simulink model "adaptive_mdl"  (R2025b)
settings: Solver=ode8  StartTime=0.0  StopTime=150  RelTol=1e-3
undefined symbols (not defined in the file): K, L0, omega, T, Tf, umax
libraries: simulink x2
settings Model: Creator=rapaja  LastModifiedBy=Predrag
settings SolverCC: AlgebraicLoopSolver=TrustRegion
settings DebuggingCC: UnconnectedInputMsg=warning  UnconnectedOutputMsg=warning  UnconnectedLineMsg=warning
settings ModelReferenceCC: EnableRefExpFcnMdlSchedulingChecks=on
settings RTWCC: GPUComputeCapability=3.5

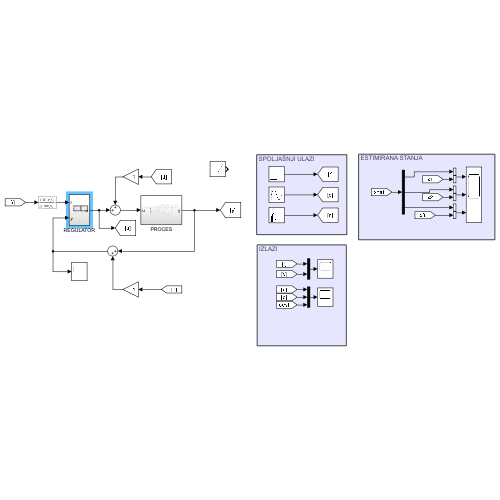
[thumbnail: Simulink's stored preview of the top-level diagram]
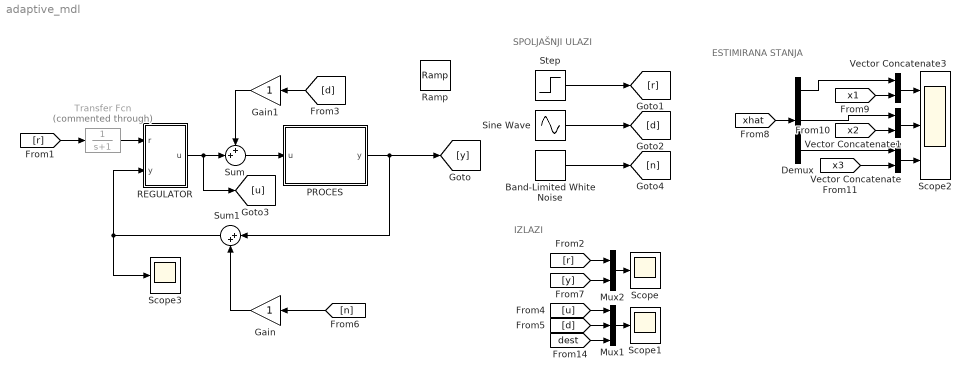
== system adaptive_mdl ==
  note: ESTIMIRANA STANJA
  note: IZLAZI
  note: SPOLJAŠNJI ULAZI
  Band-Limited White Noise : simulink/Sources/Band-Limited White Noise  Cov=[0.00001]  Ts=T  seed=[23341]
  Demux : Demux  Outputs=3
  Gain : Gain
  Gain1 : Gain
  Mux1 : Mux  Inputs=3
  Mux2 : Mux  Inputs=2
  PROCES : Subsystem
  REGULATOR : Subsystem
  Ramp : simulink/Sources/Ramp  slope=1  start=0  InitialOutput=0
  Scope : Scope
      settings: ActiveDisplayYMinimum=-7.6055878064098327E+152  ActiveDisplayYMaximum=1.3812329514646694E+152
  Scope1 : Scope
      settings: ActiveDisplayYMinimum=-4.4199585625146725  ActiveDisplayYMaximum=30.491106506946075
  Scope2 : Scope  NumInputPorts=3
      settings: ActiveDisplayYMinimum=-0.25565847863628133  ActiveDisplayYMaximum=2.1794222293336483  DataLoggingVariableName=ScopeData2
  Scope3 : Scope
      settings: ActiveDisplayYMinimum=-4.0357975554112038  ActiveDisplayYMaximum=7.5925968634709662  DataLoggingVariableName=ScopeData3
  Sine Wave : Sin  Amplitude=0.1  Frequency=omega  SampleTime=0
  Step : Step  Time=2  SampleTime=0
  Sum : Sum  Inputs=++|
  Sum1 : Sum  Inputs=|++
  Transfer Fcn : TransferFcn  Commented=through  Denominator=[1 1]
  Vector Concatenate : Concatenate
  Vector Concatenate1 : Concatenate
  Vector Concatenate3 : Concatenate
  wires:
  REGULATOR/1(u) -> Sum/2, [u]
  [d] -> Gain1/1
  Band-Limited White Noise/1 -> [n]
  Gain/1 -> Sum1/2
  Gain1/1 -> Sum/1
  [r] -> Mux2/1
  [y] -> Mux2/2
  Mux2/1 -> Scope/1
  Mux1/1 -> Scope1/1
  [u] -> Mux1/1
  [d] -> Mux1/2
  PROCES/1(y) -> Sum1/1, [y]
  Sum/1 -> PROCES/1(u)
  Sum1/1 -> Scope3/1, REGULATOR/2(y)
  Step/1 -> [r]
  [n] -> Gain/1
  [r] -> Transfer Fcn/1
  [xhat] -> Demux/1
  Vector Concatenate/1 -> Scope2/3
  Demux/3 -> Vector Concatenate/1
  [x3] -> Vector Concatenate/2
  Vector Concatenate1/1 -> Scope2/2
  Demux/2 -> Vector Concatenate1/1
  [x2] -> Vector Concatenate1/2
  Vector Concatenate3/1 -> Scope2/1
  [x1] -> Vector Concatenate3/2
  Demux/1 -> Vector Concatenate3/1
  [dest] -> Mux1/3
  Sine Wave/1 -> [d]
  Transfer Fcn/1 -> REGULATOR/1(r)

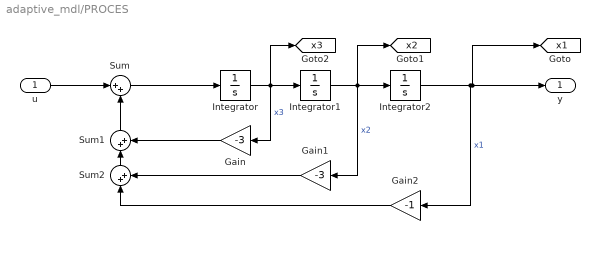
== system adaptive_mdl/PROCES ==
  u : Inport
  Gain : Gain  Gain=-3
  Gain1 : Gain  Gain=-3
  Gain2 : Gain  Gain=-1
  Integrator : Integrator
  Integrator1 : Integrator
  Integrator2 : Integrator
  Sum : Sum  Inputs=|++
  Sum1 : Sum  Inputs=|++
  Sum2 : Sum  Inputs=|++
  y : Outport
  tag scope: x1=global, x2=global, x3=global
  wires:
  Integrator2/1 -> [x1], y/1, Gain2/1  "x1"
  Integrator1/1 -> [x2], Integrator2/1, Gain1/1  "x2"
  Integrator/1 -> [x3], Integrator1/1, Gain/1  "x3"
  u/1 -> Sum/1
  Sum/1 -> Integrator/1
  Gain/1 -> Sum1/2
  Sum1/1 -> Sum/2
  Sum2/1 -> Sum1/1
  Gain1/1 -> Sum2/2
  Gain2/1 -> Sum2/1

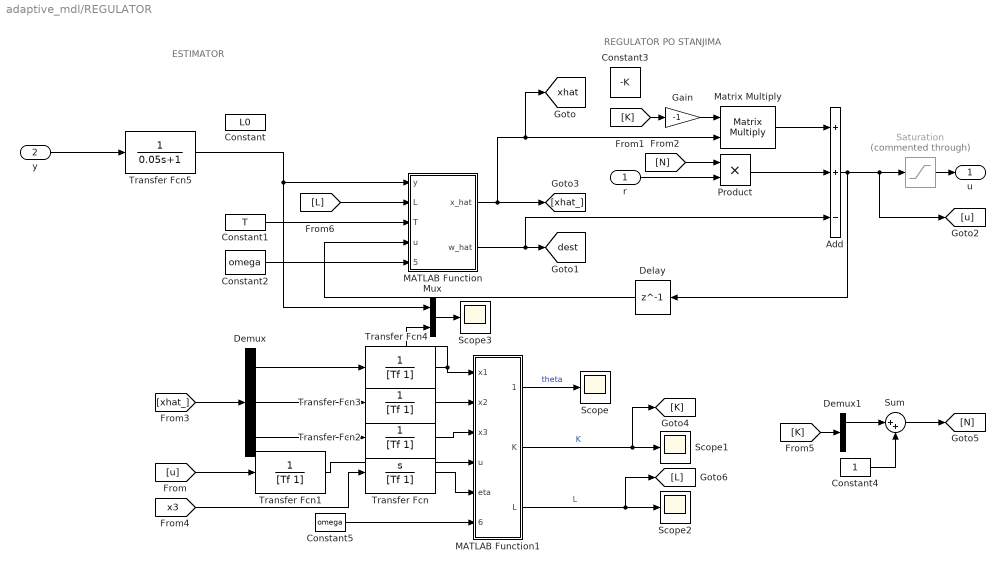
== system adaptive_mdl/REGULATOR ==
  note: REGULATOR PO STANJIMA
  note: ESTIMATOR
  r : Inport
  y : Inport  Port=2
  Add : Sum  Inputs=++-
  Constant : Constant  Value=L0  VectorParams1D=off
  Constant1 : Constant  Value=T
  Constant2 : Constant  Value=omega
  Constant3 : Constant  Value=-K  VectorParams1D=off
  Constant4 : Constant
  Constant5 : Constant  Value=omega
  Delay : Delay  DelayLength=1
  Demux : Demux  Outputs=3
  Demux1 : Demux  Outputs=3
  Gain : Gain  Gain=-1
  MATLAB Function : MATLAB Function  TreatAsAtomicUnit=on
  MATLAB Function1 : MATLAB Function  TreatAsAtomicUnit=on
  Matrix Multiply : Product  Multiplication=Matrix(*)
  Mux : Mux  Inputs=2
  Product : Product
  Saturation : Saturate  Commented=through  UpperLimit=umax  LowerLimit=-umax
  Scope{,1..3} (4 alike) : Scope
      Scope settings: ActiveDisplayYMinimum=-9.8962067879679338  ActiveDisplayYMaximum=10.094491357245289  DataLoggingVariableName=ScopeData4
      Scope1 settings: ActiveDisplayYMinimum=-9936.0105990375614  ActiveDisplayYMaximum=89991.778955448608  DataLoggingVariableName=ScopeData5
      Scope2 settings: ActiveDisplayYMinimum=-6128.36903688629  ActiveDisplayYMaximum=10361.834235959417  DataLoggingVariableName=ScopeData6
      Scope3 settings: ActiveDisplayYMinimum=-0.18469851412713539  ActiveDisplayYMaximum=1.5002818001789731  DataLoggingVariableName=ScopeData7
  Sum : Sum  Inputs=|++
  Transfer Fcn : TransferFcn  Numerator=[1 0]  Denominator=[Tf 1]
  Transfer Fcn{1..4} (4 alike) : TransferFcn  Numerator=[1 ]  Denominator=[Tf 1]
  Transfer Fcn5 : TransferFcn  Numerator=[1 ]  Denominator=[0.05 1]
  u : Outport
  tag scope: dest=global, xhat=global
  wires:
  y/1 -> Transfer Fcn5/1
  Constant1/1 -> MATLAB Function/3(T)
  MATLAB Function/1(x_hat) -> [xhat_], [xhat], Matrix Multiply/2
  MATLAB Function/2(w_hat) -> Add/3, [dest]
  Constant2/1 -> MATLAB Function/5(omega)
  Matrix Multiply/1 -> Add/1
  r/1 -> Product/2
  Delay/1 -> MATLAB Function/4(u)
  Product/1 -> Add/2
  Saturation/1 -> u/1
  Add/1 -> [u], Saturation/1, Delay/1
  MATLAB Function1/1(theta_) -> Scope/1  "theta"
  MATLAB Function1/2(K) -> [K], Scope1/1  "K"
  Transfer Fcn1/1 -> MATLAB Function1/4(u)
  Transfer Fcn2/1 -> MATLAB Function1/3(x3)
  Transfer Fcn3/1 -> MATLAB Function1/2(x2)
  Transfer Fcn4/1 -> MATLAB Function1/1(x1), Mux/2
  Demux/1 -> Transfer Fcn4/1
  Demux/2 -> Transfer Fcn3/1
  Demux/3 -> Transfer Fcn2/1
  [N] -> Product/1
  Sum/1 -> [N]
  Demux1/1 -> Sum/1
  Constant4/1 -> Sum/2
  [K] -> Demux1/1
  [K] -> Gain/1
  Gain/1 -> Matrix Multiply/1
  MATLAB Function1/3(L) -> [L], Scope2/1  "L"
  [L] -> MATLAB Function/2(L)
  [xhat_] -> Demux/1
  Transfer Fcn/1 -> MATLAB Function1/5(eta)
  Mux/1 -> Scope3/1
  [x3] -> Transfer Fcn/1
  [u] -> Transfer Fcn1/1
  Constant5/1 -> MATLAB Function1/6(omega)
  Transfer Fcn5/1 -> Mux/1, MATLAB Function/1(y)

== matlab function adaptive_mdl/REGULATOR/MATLAB Function1 ==
  settings: updateMethod=DISCRETE
  data: x1 input; x2 input; x3 input; u input; theta_ output; eta input; K output; L output; omega input
function [theta_, K, L]  = fcn(x1, x2, x3, u, eta, omega)

phi = [-x3;-x2;-x1;u];

persistent theta;
persistent P;

if(isempty(theta))
    theta = zeros(length(phi), 1) + 0.1;
end


if(isempty(P))
    P = 9999 .* eye(length(phi), length(phi));
end


P = P - (P * (phi * phi') * P) / (1 + phi' * P * phi);
eps = eta - phi' * theta;
theta = theta + (P*phi) * eps;

theta_ = theta;

b0 = theta(4, 1);
a0 = theta(3, 1);
a1 = theta(2, 1);
a2 = theta(1, 1);


%Pole placement
pk = poly(-20 * [1 1 1]);
K = zeros(1, 3);
K(1, 1) = (pk(1, 4) - a0) / b0;
K(1, 2) = (pk(1, 3) - a1) / b0;
K(1, 3) = (pk(1, 2) - a2) / b0;


p = poly(-2 * [1 1 1 1 1]);
L = zeros(1, 5);
L(1, 1) = p(1, 2) - a2;
L(1, 2) = p(1, 3) - a1 - a2*L(1, 1) - omega^2;
L(1, 3) = p(1, 4) - a0 - a1 * L(1, 1) -a2 * L(1, 2) - omega*2 * L(1, 1);
L(1, 4) = (p(1, 5) - a0 * L(1, 1) -a1 * L(1, 2) - a2*L(1, 3) - omega^2 * L(1, 2)) / b0;
L(1, 5) = (p(1, 6) - a0 * L(1, 2) -a1 * L(1, 3) - a2 * L(1, 4) - omega^2 * L(1, 3)) / b0;

== matlab function adaptive_mdl/REGULATOR/MATLAB Function ==
  settings: updateMethod=DISCRETE  sampleTime=T
  data: y input; x_hat output; L input; T input; u input; w_hat output; omega input
function [x_hat, w_hat] = fcn(y, L, T, u, omega)
persistent x1hat
persistent x2hat
persistent x3hat
persistent w1hat
persistent w2hat

if(isempty(x1hat))
    x1hat = 0;
end
if(isempty(x2hat))
    x2hat = 0;
end
if(isempty(x3hat))
    x3hat = 0;
end
if(isempty(w1hat))
    w1hat = 0;
end
if(isempty(w2hat))
    w2hat = 0;
end
e = y - x1hat;

x1hat_n = x1hat + T * (x2hat + L(1, 1) * e);
x2hat_n = x2hat + T * (x3hat + L(1, 2) * e);
x3hat_n = x3hat + T * (-3*x3hat - 3*x2hat -x1hat + u + w1hat + L(1, 3) * e);
w1hat_n = w1hat + T * ( w2hat + L(1, 4) * e);
w2hat_n = w2hat + T * (-omega^2 * w1hat +  L(1, 5) * e);

x1hat = x1hat_n;
x2hat = x2hat_n;
x3hat = x3hat_n;
w1hat = w1hat_n;
w2hat = w2hat_n;

x_hat = [x1hat; x2hat; x3hat];
w_hat = w1hat;
